simulink library "mode_select_lib"  (R2018b)
settings: Solver=VariableStepAuto  StartTime=0.0  StopTime=10.0  RelTol=1e-3
undefined symbols (not defined in the file or in its folder): fswParams
libraries: simulink x1, two_norm x1, desat_timer_logic_lib x1
settings Model: Creator=colem  LastModifiedBy=colem

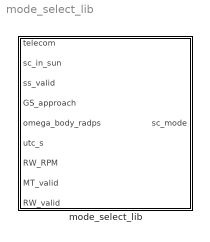
== system mode_select_lib ==
  mode_select_lib : Subsystem

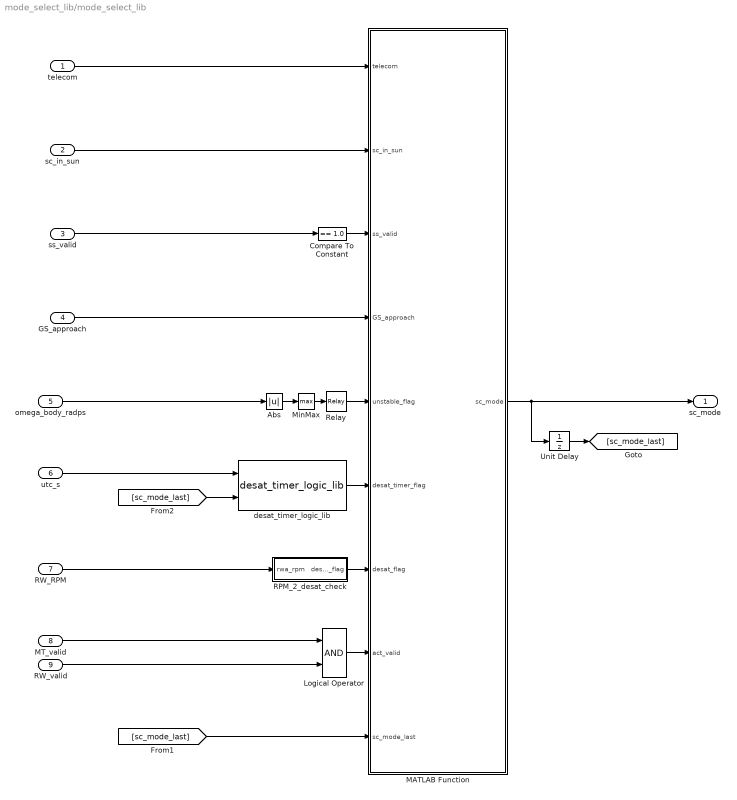
== system mode_select_lib/mode_select_lib ==
  telecom : Inport
  sc_in_sun : Inport  Port=2
  ss_valid : Inport  Port=3
  GS_approach : Inport  Port=4
  omega_body_radps : Inport  Port=5
  utc_s : Inport  Port=6
  RW_RPM : Inport  Port=7
  MT_valid : Inport  Port=8
  RW_valid : Inport  Port=9
  Abs : Abs
  Compare To Constant : simulink/Logic and Bit Operations/Compare To Constant  relop===  const=1.0  OutDataTypeStr=boolean
  Logical Operator : Logic  AllPortsSameDT=off  OutDataTypeStr=boolean
  MATLAB Function : MATLAB Function  TreatAsAtomicUnit=on
  MinMax : MinMax  Function=max
  RPM_2_desat_check : Subsystem
  Relay : Relay  OnSwitchValue=fswParams.mode_select.body_rate_threshold_max  OffSwitchValue=fswParams.mode_select.body_rate_threshold_min
  Unit Delay : UnitDelay  InitialCondition=fswParams.mode_select.sc_mode_ic  SampleTime=-1
  desat_timer_logic_lib : desat_timer_logic_lib/desat_timer_logic_lib  SystemSampleTime=-1
  sc_mode : Outport
  wires:
  ss_valid/1 -> Compare To Constant/1
  telecom/1 -> MATLAB Function/1(telecom)
  MT_valid/1 -> Logical Operator/1
  Abs/1 -> MinMax/1
  MinMax/1 -> Relay/1
  Compare To Constant/1 -> MATLAB Function/3(ss_valid)
  omega_body_radps/1 -> Abs/1
  GS_approach/1 -> MATLAB Function/4(GS_approach)
  sc_in_sun/1 -> MATLAB Function/2(sc_in_sun)
  RW_valid/1 -> Logical Operator/2
  Logical Operator/1 -> MATLAB Function/8(act_valid)
  Unit Delay/1 -> [sc_mode_last]
  MATLAB Function/1(sc_mode) -> Unit Delay/1, sc_mode/1
  RPM_2_desat_check/1(desat_flag) -> MATLAB Function/7(desat_flag)
  [sc_mode_last] -> MATLAB Function/9(sc_mode_last)
  Relay/1 -> MATLAB Function/5(unstable_flag)
  desat_timer_logic_lib/1 -> MATLAB Function/6(desat_timer_flag)
  utc_s/1 -> desat_timer_logic_lib/1
  RW_RPM/1 -> RPM_2_desat_check/1(rwa_rpm)
  [sc_mode_last] -> desat_timer_logic_lib/2

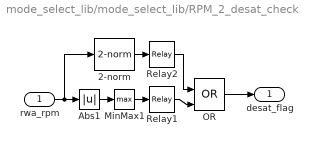
== system mode_select_lib/mode_select_lib/RPM_2_desat_check ==
  rwa_rpm : Inport
  2-norm : two_norm/2-norm  SystemSampleTime=-1
  Abs1 : Abs
  MinMax1 : MinMax  Function=max
  OR : Logic  Operator=OR  IconShape=distinctive  AllPortsSameDT=off  OutDataTypeStr=boolean
  Relay1 : Relay  OnSwitchValue=fswParams.mode_select.RWA_RPM_threshold_max_inf  OffSwitchValue=fswParams.mode_select.RWA_RPM_threshold_min_inf
  Relay2 : Relay  OnSwitchValue=fswParams.mode_select.RWA_RPM_threshold_max_2norm  OffSwitchValue=fswParams.mode_select.RWA_RPM_threshold_min_2norm
  desat_flag : Outport
  wires:
  Relay2/1 -> OR/1
  rwa_rpm/1 -> Abs1/1, 2-norm/1
  MinMax1/1 -> Relay1/1
  Relay1/1 -> OR/2
  2-norm/1 -> Relay2/1
  Abs1/1 -> MinMax1/1
  OR/1 -> desat_flag/1

== matlab function mode_select_lib/MATLAB Function ==
  data: telecom input; sc_mode output; sc_in_sun input; ss_valid input; GS_approach input; unstable_flag input; desat_timer_flag input; desat_flag input; act_valid input; sc_mode_last input int8
% Logic for selecting the gnc operating mode
%
% Author: Cole Morgan 7.8.19
%
% modelled after RAIN-SAT -- T. Reynolds 2.15.18



function sc_mode  = mode_logic(telecom,sc_in_sun,ss_valid,GS_approach, unstable_flag, desat_timer_flag, ...
    desat_flag, act_valid, sc_mode_last)

%GNC_MODE_LOGIC    GNC Mode Selector
%
% Chooses control mode based on sensor and actuator data.
%   mode_logic.low_power        = 1; "safe mode"
%   mode_logic.idle             = 2; "idle/standby mode"
%   mode_logic.stabilize        = 3;
%   mode_logic.nominal          = 4;
%       nominal.desat           = 41;
%       nominal.sun_seek        = 42;
%   mode_logic.point            = 5;
%       point.com               = 51;
%       point.image             = 52;
%       point.exp               = 53;
%
% ----- INPUTS -----
%
% 1. telecom - Data coming from the bus. Parsed according to:
%
%   telecom(1) == Override the autonomous mode selection and command the mode
%               corresponding to this number. Set to 0 if the autonomous 
%               selection is to go ahead. Type: int8
%   telecom(2) == Reboot just occured OR we just exited a detumble. 
%               s/c will sit in this mode until either pointing takes over
%               or body rates rise again. Type: int8
%   telecom(3) == Go ahead for the pointing mode. One means the s/c
%               is go for pointing of any kind. Type: int8
% 
%   telecom(4) == Low power mode is enforced. only sgp4 on
%
%   telecom(5) == Idle mode is enforced. actuators and sensors have power,
%   but no actuator/control signals are sent. check status.
%
%   telecom(6) == Requesting an image.
%
%   telecom(7) == Allow GNC-2 from ground command.
%
% 2. sc_in_sun: - Tells us if the s/c is in eclipse. Type: boolean.
% 3. ss_valid:  - validity bit from the sun_sensor. Used to decide if we
%                   need to enter sun_seek mode
% 4. gs_appraoch: - Tells us if the ground station is approaching based on
%                   reorientation criteria. Type: boolean.
%
% stable_flag: - Rates are all below some threshold that defines stability.
% essentially not spinning. Goes low when tumbling.
%
% desat_flag: - Goes high when thresh_max is hit, and does not go low until 
% thresh_min is hit (hysteresis). Uses reaction wheel RPM thresholds.
%
% low_power_flag: - This should maybe be a telecom condition. used to
% enforce low power throughout sc
%
% sc_mode_old - Previous spacecraft state, used to test exit conditions for
%                   each mode.
%
% ----- OUTPUTS -----
%
% sc_mode - Spacecraft state determined. Type: double.
%
% sc_exp - Extra state corresponding to what type of experimental control
%           is engaged. Only nonzero if sc_mode == 33.



% Default to last known condition and no experimental control
sc_mode     = int8(sc_mode_last);

if( telecom(4) == 1)
    sc_mode = int8(1.0);
    % This has high priority. Power actuators and sensors off. leave only sgp4 on. 
    return;
    
elseif( telecom(5) == 1 || (~act_valid))
    sc_mode = int8(2.0);
    % This has high priority. Power actuators and sensors on. start estimating attiude and diagnosing 
    % hardware health but dont send control commands.
    return;

    
    %at this point nothing important is being enforced. always default to stabilizing
    %then sun pointing.
elseif( telecom(1) == 0 )
    
    
    %check if you are stable and not trying to point. stable flag needs to be a threshold band. 
    if( unstable_flag == 1) %&& telecom(3) ~= 1) % sc_mode_last <= 3 
        sc_mode = int8(3.0);
        if (sc_mode_last == 41.0)
            sc_mode = int8(41.0);
%             if(desat_timer_flag == 0)
%                 sc_mode = int8(3.0);
%             end
        end
        %If unstable, first stabilize sc.
        return;
    end
    
    % by this point, sc is in nominal mode
    
    %Check if motors are saturated
    if(desat_flag || desat_timer_flag)
        if(~desat_flag)
            sc_mode = int8(3.0);
                % the timer was triggered, but you don't need to desat.
                % wait in ASM until timer goes down.
        else
            sc_mode = int8(41.0);
                % if you need to desat, desat.
        end
        return;
        %If motors are saturated, desaturate.
    end
    
    % If we are not in Earth's shadow but the sun_sensor is reporting
    % invalid, then we need to move to acquire the sun in the FoV of the
    % sun_sensor. Hence enter sun_seek mode.
    if( sc_in_sun && ~ss_valid )
       sc_mode  = int8(42.0);
       %return;
    end
    
    
    % If all cases upstream have been passed, then enter pointing mode if
    % allowed to do so. Check for pointing condition from CAN
    if( telecom(3) == 1 )
        % Default to communication pointing mode
        sc_mode     = int8(51.0);
        
        % Check to see if entering GS range and not in eclipse and an image
        % was requested
        if( GS_approach && sc_in_sun && telecom(6) == 1 )
            sc_mode  = int8(52.0);
        end
        
        % Check to see if experiment was requested. 
        if( telecom(7) == 1 )
            sc_mode  = int8(53.0);
        end
        
    end
    
% If signal received to override the autonomous mode selection, set mode 
% based on CAN(1) value.
elseif( telecom(1) ~= 0 )
    
    sc_mode = int8(telecom(1));
    
end
